simulink model "LCLR_PI_Stablized"  (R2017a)
settings: Solver=ode1  StartTime=0.0  StopTime=0.1  FixedStep=Ts_Pw  RelTol=1e-3
InitFcn:
  | clc;
  | clear all;
  | Ts_Control=1e-4;
  | Ts_Pw=1e-7;
  | Ts_Sc=30*Ts_Pw;
  | h=Ts_Control;
  | 
  | L1= 3.87e-3 ;
  | L2 = 2.4e-3 ;
  | C= 10e-6 ;
  | rC = 2.78 ;
undefined symbols (not defined in the file): DiscIntNeverNeededParam
libraries: powerlib x10, powerlib_extras x3, simulink x1
settings Model: ExtModeTrigDuration=5000  Creator=Administrator  LastModifiedBy=donghao
settings SolverCC: PositivePriorityOrder=on
settings DataIOCC: LimitDataPoints=on  SaveFormat=Array  SignalLoggingSaveFormat=ModelDataLogs
settings OptimizationCC: ExpressionDepthLimit=2147483647  InitFltsAndDblsToZero=on  LifeSpan=inf
settings DebuggingCC: UnderspecifiedInitializationDetection=Classic  MergeDetectMultiDrivingBlocksExec=none  SolverPrmCheckMsg=warning  FcnCallInpInsideContextMsg=warning  UnconnectedInputMsg=none  UnconnectedOutputMsg=none  UnconnectedLineMsg=none  StateNameClashWarn=warning  SFUnexpectedBacktrackingDiag=warning  SFNoUnconditionalDefaultTransitionDiag=warning  SFExecutionAtInitializationDiag=none
settings HardwareCC: ProdBitPerPointer=32  ProdBitPerSizeT=32  ProdBitPerPtrDiffT=32  ProdLargestAtomicFloat=None  ProdIntDivRoundTo=Undefined  ProdEndianess=Unspecified  ProdWordSize=32  ProdHWDeviceType=32-bit Generic
settings ModelReferenceCC: PropagateSignalLabelsOutOfModel=off
settings RTWCC: SystemTargetFile=quarc_windows.tlc  TemplateMakefile=quarc_default_tmf  Description=QUARC Win32 Target
settings STFCustomTargetCC: TargetPreCompLibLocation=C:\DOCUME~1\ALLUSE~1\APPLIC~1\QUARC\lib\2007b\windows\release  GeneratePreprocessorConditionals=Disable all  CPPClassGenCompliant=on  SystemTargetFile=quarc_windows.tlc
settings GRTTargetCC: TargetPreCompLibLocation=C:\DOCUME~1\ALLUSE~1\APPLIC~1\QUARC\lib\2007b\windows\release  TargetLangStandard=C89/C90 (ANSI)  ParMdlRefBuildCompliant=off  CompOptLevelCompliant=off  ConcurrentExecutionCompliant=off  GeneratePreprocessorConditionals=Disable all  CombineOutputUpdateFcns=off  MatFileLogging=off  GRTInterface=on  UseToolchainInfoCompliant=off  ExtMode=on  ExtModeMexFile=noextcomm
settings ConfigComp: CovMetricSettings=dw  CovHtmlReporting=on  CovSaveCumulativeToWorkspaceVar=on  CovSaveSingleToWorkspaceVar=on  CovExternalEMLEnable=off

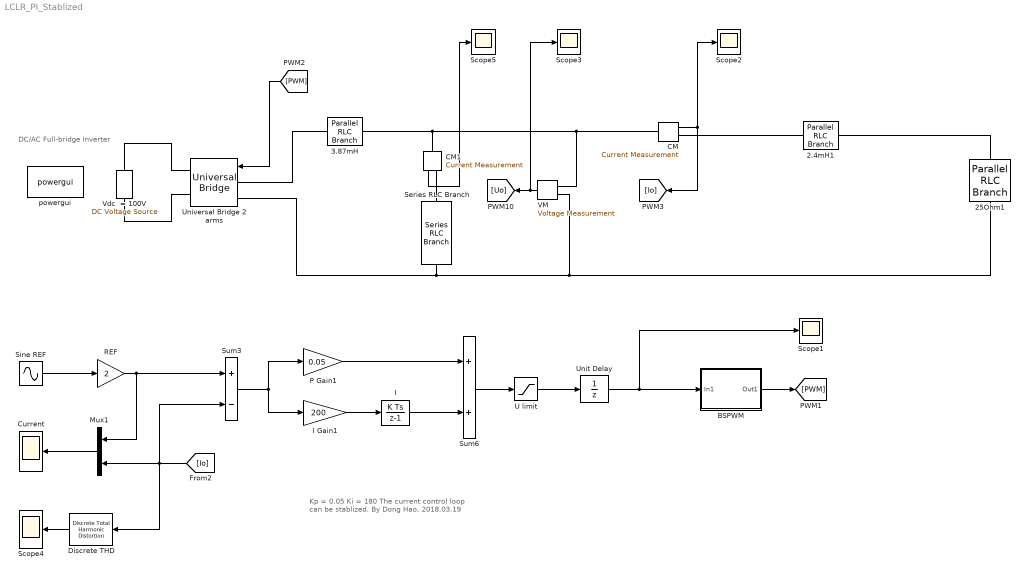
== system LCLR_PI_Stablized ==
  note: DC/AC Full-bridge
      | Inverter
  note: Kp = 0.05
      | Ki = 180
      | The current control loop can be stablized.
      | By Dong Hao, 2018.03.19
  2.4mH1 : powerlib/Elements/Parallel RLC Branch  LConnTagsString=a  RConnTagsString=__new0  BranchType=L  Resistance=1.0  Inductance=L2  SetiL0=off  InitialCurrent=0  Capacitance=1.0  Setx0=off  InitialVoltage=0  Measurements=Branch voltage and current
  25Ohm1 : powerlib/Elements/Parallel RLC Branch  LConnTagsString=a  RConnTagsString=__new0  BranchType=R  Resistance=25  Inductance=0.002  SetiL0=off  InitialCurrent=0  Capacitance=16e-6  Setx0=off  InitialVoltage=0  Measurements=Branch voltage and current
  3.87mH : powerlib/Elements/Parallel RLC Branch  LConnTagsString=a  RConnTagsString=__new0  BranchType=L  Resistance=1.0  Inductance=L1  SetiL0=off  InitialCurrent=0  Capacitance=1.0  Setx0=off  InitialVoltage=0  Measurements=Branch voltage and current
  BSPWM : Subsystem
  CM : powerlib/Measurements/Current Measurement  PhasorSimulation=off  OutputType=Complex  PSBequivalent=0
  CM1 : powerlib/Measurements/Current Measurement  PhasorSimulation=off  OutputType=Complex  PSBequivalent=0
  Current : Scope
  Discrete THD : powerlib_extras/Discrete Measurements/Discrete Total Harmonic Distortion  Freq=50  Ts=Ts_Sc
  I : DiscreteIntegrator  gainval=1  SampleTime=Ts_Control  UpperSaturationLimit=+10  LowerSaturationLimit=-10  ICPrevOutput=DiscIntNeverNeededParam  ICPrevScaledInput=DiscIntNeverNeededParam
  I Gain1 : Gain  Gain=200  SaturateOnIntegerOverflow=on  OutDataTypeStr=Inherit: Same as input  ParamDataTypeStr=Inherit: Same as input
  Mux1 : Mux  Inputs=2
  P Gain1 : Gain  Gain=0.05  SaturateOnIntegerOverflow=on  OutDataTypeStr=Inherit: Same as input  ParamDataTypeStr=Inherit: Same as input
  REF : Gain  Gain=2  SaturateOnIntegerOverflow=on  OutDataTypeStr=Inherit: Same as input  ParamDataTypeStr=Inherit: Same as input
  Scope{1..5} (5 alike) : Scope
      Scope2 settings: RequirementInfo="{}  %GIDa_6a932280_eb71_47a1_a161_fcf0b45dd7b5"
  Series RLC Branch : powerlib/Elements/Series RLC Branch  LConnTagsString=__new0  RConnTagsString=__new0  BranchType=RC  Resistance=rC  Inductance=1e-3  SetiL0=off  InitialCurrent=0  Capacitance=C  Setx0=off  InitialVoltage=0  Measurements=None
  Sine REF : Sin  Frequency=2*pi*50
  Sum3 : Sum  Inputs=+-  SaturateOnIntegerOverflow=on  InputSameDT=on  OutDataTypeStr=Inherit: Same as first input
  Sum6 : Sum  SaturateOnIntegerOverflow=on  InputSameDT=on  OutDataTypeStr=Inherit: Same as first input
  U limit : Saturate  UpperLimit=1  LowerLimit=-1
  Unit Delay : UnitDelay  SampleTime=Ts_Control
  Universal Bridge 2 arms : powerlib/Power Electronics/Universal Bridge  RequirementInfo="{}  %GIDa_113e3af2_c0e9_4636_9976_9b36552fa242"  Arms=2  SnubberResistance=1e3  SnubberCapacitance=1e-6  Device=IGBT / Diodes  Ron=1e-4  Lon=0  ForwardVoltages="[  1  1  ]"  ForwardVoltage=.8  GTOparameters=[ 10e-6 , 20e-6 ]  IGBTparameters=[ 1e-6 , 2e-6 ]  Measurements=UAB UBC UCA UDC voltages  Measurements_2=None  converterType=Rectifier
  VM : powerlib/Measurements/Voltage Measurement  PhasorSimulation=off  OutputType=Complex  PSBequivalent=0
  "Vdc  = 100V  " : powerlib/Electrical Sources/DC Voltage Source  Description=source block  Amplitude=100  Measurements=None
      settings: AttributesFormatString=\n
  powergui : powerlib/powergui  SimulationMode=Discrete  SampleTime=Ts_Pw  frequency=60  Iterations=50  frequencyindice=0  Pbase=100e6  ErrMax=1e-4  UnitsV=kV  UnitsW=MW  buscounter=0  FunctionMessages=off  echomessages=off  EnableUseOfTLC=off  CurrentSourceSwitches=off  DisableSnubberDevices=off  DisableRonSwitches=off  DisableVfSwitches=off  DisplayEquations=off  SolverType=Tustin  Interpol=off  ExternalGateDelay=off  methode=off  Ts=0  x0status=blocks  SPID=off  SwTol=0  HookPort=off  RestoreLinks=warning  ResistiveCurrentMeasurement=off  Frange=[0:2:500]  Ylog=off  Xlog=on  ShowGrid=off  save=off  variable=ZData  structure=ScopeData  ZoomFFT=off  StartTime=0.04  cycles=3  DisplayStyle=1  fundamental=50  FreqAxis=off  MaxFrequency=1000  frequencyindicesteady=1  RmsSteady=1  display=off
  wires:
  REF/1 -> Mux1/1, Sum3/1
  U limit/1 -> Unit Delay/1
  Sine REF/1 -> REF/1
  [PWM] -> Universal Bridge 2 arms/1
  CM1/1 -> Scope5/1
  CM/1 -> [Io], Scope2/1
  Mux1/1 -> Current/1
  BSPWM/1(Out1) -> [PWM]
  [Io] -> Mux1/2, Discrete THD/1, Sum3/2
  VM/1 -> Scope3/1, [Uo]
  Discrete THD/1 -> Scope4/1
  Unit Delay/1 -> Scope1/1, BSPWM/1(In1)
  Sum6/1 -> U limit/1
  I Gain1/1 -> I/1
  P Gain1/1 -> Sum6/1
  I/1 -> Sum6/2
  Sum3/1 -> I Gain1/1, P Gain1/1
  connections:
  Series RLC Branch/RConn1 -- Universal Bridge 2 arms/LConn2 -- VM/LConn2 -- 25Ohm1/RConn1
  Universal Bridge 2 arms/RConn2 -- "Vdc  = 100V  "/LConn1
  "Vdc  = 100V  "/RConn1 -- Universal Bridge 2 arms/RConn1
  VM/LConn1 -- CM/LConn1 -- 3.87mH/RConn1 -- CM1/LConn1
  3.87mH/LConn1 -- Universal Bridge 2 arms/LConn1
  Series RLC Branch/LConn1 -- CM1/RConn1
  CM/RConn1 -- 2.4mH1/LConn1
  25Ohm1/LConn1 -- 2.4mH1/RConn1

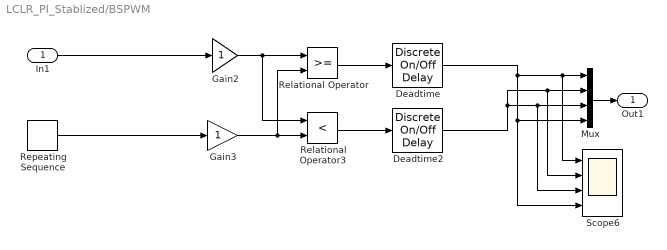
== system LCLR_PI_Stablized/BSPWM ==
  In1 : Inport
  Deadtime : powerlib_extras/Discrete  Control Blocks/Discrete On//Off Delay  type_delay=On delay  delay=3e-6  ic=0  Ts=Ts_Pw
  Deadtime2 : powerlib_extras/Discrete  Control Blocks/Discrete On//Off Delay  type_delay=On delay  delay=3e-6  ic=0  Ts=Ts_Pw
  Gain2 : Gain
  Gain3 : Gain  SampleTime=Ts_Pw
  Mux : Mux
  Relational Operator : RelationalOperator  OutDataTypeStr=boolean  SampleTime=Ts_Pw  RndMeth=Nearest
  Relational Operator3 : RelationalOperator  Operator=<  OutDataTypeStr=boolean  SampleTime=Ts_Pw  RndMeth=Nearest
  Repeating Sequence : simulink/Sources/Repeating Sequence  rep_seq_t="[0 Ts_Control/4 Ts_Control/2 3*Ts_Control/4  Ts_Control]"  rep_seq_y=[0 1 0 -1 0]
  Scope6 : Scope  NumInputPorts=4
  Out1 : Outport
  wires:
  Mux/1 -> Out1/1
  Gain3/1 -> Relational Operator/2, Relational Operator3/2
  Deadtime/1 -> Mux/1, Scope6/1, Mux/4, Scope6/4
  Relational Operator/1 -> Deadtime/1
  Repeating Sequence/1 -> Gain3/1
  Relational Operator3/1 -> Deadtime2/1
  Deadtime2/1 -> Mux/2, Scope6/2, Mux/3, Scope6/3
  In1/1 -> Gain2/1
  Gain2/1 -> Relational Operator/1, Relational Operator3/1
